simulink model "a8"  (R2021a)
settings: Solver=VariableStepAuto  StartTime=0.0  StopTime=3  RelTol=1e-3
undefined symbols (not defined in the file or in its folder): Down, Ion, Lithium, Up
libraries: spsCurrentMeasurementLib x22, spsVoltageMeasurementLib x17, spsSeriesRLCBranchLib x11, spsGroundLib x6, powerlib_extras x4, spsACVoltageSourceLib x3, spsIGBTDiodeLib x3, dspsigops x3, spsPower3phInstantaneousLib x3, spsDiodeLib x2, spsUniversalBridgeLib x2, spsBatteryLib x1
(part 1 of 2)
settings Model: Creator=Dell  LastModifiedBy=Dell
settings SolverCC: ZeroCrossControl=DisableAll
settings DebuggingCC: ModelReferenceExtraNoncontSigs=none

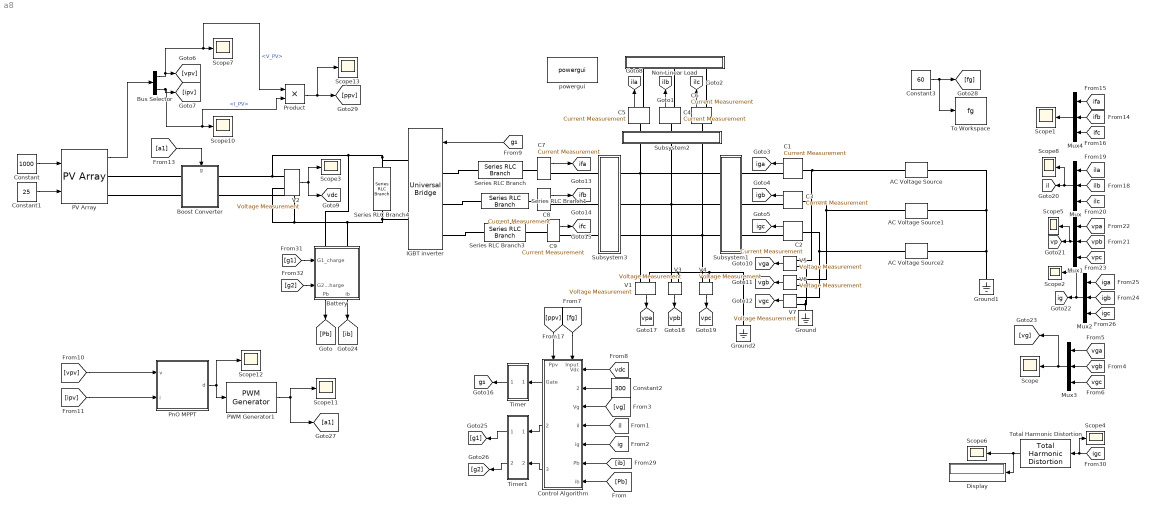
== system a8 ==
  AC Voltage Source : spsACVoltageSourceLib/AC Voltage Source  Amplitude=230  Phase=0  Frequency=60  SampleTime=0  Measurements=None  BusType=swing  Pref=10e3  Qref=0  Qmin=-inf  Qmax=+inf
  AC Voltage Source1 : spsACVoltageSourceLib/AC Voltage Source  Amplitude=230  Phase=120  Frequency=60  SampleTime=0  Measurements=None  BusType=swing  Pref=10e3  Qref=0  Qmin=-inf  Qmax=+inf
  AC Voltage Source2 : spsACVoltageSourceLib/AC Voltage Source  Amplitude=230  Phase=-120  Frequency=60  SampleTime=0  Measurements=None  BusType=swing  Pref=10e3  Qref=0  Qmin=-inf  Qmax=+inf
  Battery : Subsystem
      settings: PortSchema="{\"entries\":[{\"content\":{\"sides\":[{\"content\":{\"connectorIds\":[\"LConn1\",\"LConn2\"]},\"type\":\"ConnectorPlacement.EquallySpacedRectSide\",\"uuid\":\"3f024d4f-4944-46f1-a681-19b9b6f5c2e3\"},{\"content\":{\"connectorIds\":[\"Out1\",\"Out2\"],\"side\":\"RIGHT\"},\"type\":\"ConnectorPlacement.EquallySpacedRectSide\",\"uuid\":\"ba9189b8-b241-4d0f-92c2-ffae32477602\"},{\"content\":{\"connectorIds\":[\"In1\",\"In2\"],\"side\":\"TOP\"},\"type\":\"ConnectorPlacement.EquallySpacedRectSide\",\"uuid\":\"2b5a68b6-4f88-4313-be0a-70c6e84ce948\"}]},\"type\":\"ConnectorPlacement.EquallySpacedConnector\",\"uuid\":\"57f7ac83-2601-4f06-be16-46ca99d36a1f\"}],\"packageUris\":[\"http://schema.mathworks.com/mf0/Connector/R2020b\"],\"version\":\"1.0\"}"
  Boost Converter : Subsystem
      settings: PortSchema="{\"entries\":[{\"content\":{\"sides\":[{\"content\":{\"connectorIds\":[\"LConn1\",\"LConn2\"]},\"type\":\"ConnectorPlacement.EquallySpacedRectSide\",\"uuid\":\"8d150eef-90b5-4fdb-be84-a9f6f4ebd895\"},{\"content\":{\"connectorIds\":[\"RConn1\",\"RConn2\"],\"side\":\"RIGHT\"},\"type\":\"ConnectorPlacement.EquallySpacedRectSide\",\"uuid\":\"8602e169-ea88-4412-9b25-fadbb117dfcf\"},{\"content\":{\"connectorIds\":[\"In1\"],\"side\":\"TOP\"},\"type\":\"ConnectorPlacement.EquallySpacedRectSide\",\"uuid\":\"8809c1af-ab1c-4eed-b81f-f8f2792471ea\"}]},\"type\":\"ConnectorPlacement.EquallySpacedConnector\",\"uuid\":\"c77f0f7f-21b7-47e6-a535-29cdb02ea9e2\"}],\"packageUris\":[\"http://schema.mathworks.com/mf0/Connector/R2020b\"],\"version\":\"1.0\"}"
  Bus Selector : BusSelector  OutputSignals=V_PV,I_PV
  C{1..9} (9 alike) : spsCurrentMeasurementLib/Current Measurement  PhasorSimulation=off  OutputType=Complex  PSBequivalent=0
  Constant : Constant  Value=1000
  Constant1 : Constant  Value=25
  Constant2 : Constant  Value=300
  Constant3 : Constant  Value=60
  Control Algorithm : Subsystem
      settings: PortSchema="{\"entries\":[{\"content\":{\"sides\":[{\"content\":{\"connectorIds\":[\"In1\",\"In2\",\"In3\",\"In4\",\"In5\",\"In6\",\"In7\"]},\"type\":\"ConnectorPlacement.EquallySpacedRectSide\",\"uuid\":\"49955e1e-2d38-4dcf-bb6a-38e771f1236c\"},{\"content\":{\"connectorIds\":[\"Out1\",\"Out2\",\"Out3\"],\"side\":\"RIGHT\"},\"type\":\"ConnectorPlacement.EquallySpacedRectSide\",\"uuid\":\"694b0366-9509-4aa0-9deb-ec901696235e\"},{\"content\":{\"connectorIds\":[\"In8\",\"In9\"],\"side\":\"TOP\"},\"type\":\"ConnectorPlacement.EquallySpacedRectSide\",\"uuid\":\"46f645d8-58d8-49b1-a06d-69f87343fd2f\"}]},\"type\":\"ConnectorPlacement.EquallySpacedConnector\",\"uuid\":\"9b034317-3015-420d-970f-6f1221e48493\"}],\"packageUris\":[\"http://schema.mathworks.com/mf0/Connector/R2020b\"],\"version\":\"1.0\"}"
  Display : Display
  Ground : spsGroundLib/Ground  LConnTagsString=a
  Ground1 : spsGroundLib/Ground  LConnTagsString=a
  Ground2 : spsGroundLib/Ground  LConnTagsString=a
  IGBT inverter : spsUniversalBridgeLib/Universal Bridge  Arms=3  SnubberResistance=1e5  SnubberCapacitance=inf  Device=IGBT / Diodes  Ron=1e-3  Lon=0  ForwardVoltages="[  0  0  ]"  ForwardVoltage=0  GTOparameters=[ 10e-6 , 20e-6 ]  IGBTparameters=[ 1e-6 , 2e-6 ]  Measurements=Device voltages  Measurements_2=None  converterType=Rectifier
  Mux{,1..4} (5 alike) : Mux  Inputs=3
  Non-Linear Load : Subsystem
  PV Array : spsPVArrayLib/PV Array  Npar=1  Nser=6  PlotType=array @ 1000 W/m2 & specified temperatures  S_vec="[ 1000  500  100 ]"  Temp_C_vec="[ 25  ]"  ModuleName=User-defined  PlotWhenSelected=off  Pm=335.28  Ncell=60  Voc=46.8  Isc=9.3  Vm=38.1  Im=8.8  beta_Voc_pc=-0.36099  alpha_Isc_pc=0.102  beta_Voc=-0.16894  alpha_Isc=0.009486  IL=9.3302  I0=3.4457e-10  nI=1.2642  Rsh=710.4206  Rs=0.33548  RobustModel=off  RobustCellTemperature=313.3991  BAL=on  Tc=1e-6  Tfilter=5e-5
  PWM Generator1 : eePwmGenerator/PWM Generator  CarrCount=Up-Down  Tper=1/10000  Ts=5e-6
  PnO MPPT : MATLAB Function  TreatAsAtomicUnit=on
  Product : Product
  Scope{,1..8,10..13} (13 alike) : Scope
  Series RLC Branch : spsSeriesRLCBranchLib/Series RLC Branch  LConnTagsString=__new0  RConnTagsString=__new0  BranchType=L  Resistance=1  Inductance=5e-3  SetiL0=off  InitialCurrent=0  Capacitance=1e-6  Setx0=off  InitialVoltage=0  Measurements=None
  Series RLC Branch1 : spsSeriesRLCBranchLib/Series RLC Branch  LConnTagsString=__new0  RConnTagsString=__new0  BranchType=L  Resistance=1  Inductance=5e-3  SetiL0=off  InitialCurrent=0  Capacitance=1e-6  Setx0=off  InitialVoltage=0  Measurements=None
  Series RLC Branch3 : spsSeriesRLCBranchLib/Series RLC Branch  LConnTagsString=__new0  RConnTagsString=__new0  BranchType=L  Resistance=1  Inductance=5e-3  SetiL0=off  InitialCurrent=0  Capacitance=1e-6  Setx0=off  InitialVoltage=0  Measurements=None
  Series RLC Branch4 : spsSeriesRLCBranchLib/Series RLC Branch  LConnTagsString=__new0  RConnTagsString=__new0  BranchType=C  Resistance=1  Inductance=5e-3  SetiL0=off  InitialCurrent=0  Capacitance=1100e-6  Setx0=off  InitialVoltage=300  Measurements=None
  Subsystem1 : Subsystem
  Subsystem2 : Subsystem
  Subsystem3 : Subsystem
  Timer : Subsystem
  Timer1 : Subsystem
  To Workspace : ToWorkspace  VariableName=fg  SampleTime=-1
      settings: Save2DSignal=2-D array (concatenate along first dimension)
  Total Harmonic Distortion : eeTotalHarmonicDistorsion/Total Harmonic Distortion  f=50  Ts=-1
      settings: SourceProductBaseCode=PS
  V{1..7} (7 alike) : spsVoltageMeasurementLib/Voltage Measurement  PhasorSimulation=off  OutputType=Complex  PSBequivalent=0
  powergui : spspowerguiLib/powergui  Priority=1  SimulationMode=Discrete  SampleTime=5e-6  frequency=60  Iterations=50  frequencyindice=0  Pbase=100e6  ErrMax=1e-4  UnitsV=kV  UnitsW=MW  buscounter=0  FunctionMessages=off  echomessages=off  EnableUseOfTLC=off  CurrentSourceSwitches=off  DisableSnubberDevices=off  DisableRonSwitches=off  DisableVfSwitches=off  DisplayEquations=off  AutomaticDiscreteSolvers=off  SolverType=Tustin/Backward Euler (TBE)  Interpol=off  ExternalGateDelay=off  methode=off  Ts=100  x0status=blocks  SPID=on  SwTol=0  HookPort=off  NonlinearTolerance=1e-4  nMaxIteration=100  ContinueOnMaxIteration=off  RestoreLinks=warning  ResistiveCurrentMeasurement=off  Frange=[0:2:500]  Ylog=off  Xlog=on  ShowGrid=off  save=off  variable=ZData  structure=0  ZoomFFT=off  StartTime=0.0  cycles=1  DisplayStyle=1  fundamental=60  FreqAxis=off  MaxFrequency=1000  frequencyindicesteady=1  RmsSteady=1  display=off
  tag scope: gs=global, ifa=global, ifb=global, ifc=global, ig=global, iga=global, igb=global, igc=global, il=global, ila=global, ilb=global, ilc=global, vdc=global, vga=global, vgb=global, vgc=global, vp=global, vpa=global, vpb=global, vpc=global
  wires:
  Constant/1 -> PV Array/1
  Constant1/1 -> PV Array/2
  V2/1 -> [vdc], Scope3/1
  [g2] -> Battery/2(G2_discharge)
  Battery/2(ib) -> [ib]
  [g1] -> Battery/1(G1_charge)
  Battery/1(Pb) -> [Pb]
  V3/1 -> [vpb]
  V1/1 -> [vpa]
  V4/1 -> [vpc]
  V7/1 -> [vgc]
  V5/1 -> [vga]
  V6/1 -> [vgb]
  C1/1 -> [iga]
  C3/1 -> [igb]
  C2/1 -> [igc]
  [vgb] -> Mux3/2
  Mux3/1 -> [vg], Scope/1
  [vga] -> Mux3/1
  [vgc] -> Mux3/3
  Mux4/1 -> Scope1/1
  Total Harmonic Distortion/1 -> Scope6/1, Display/1
  [ila] -> Mux/1
  [ilb] -> Mux/2
  [vpc] -> Mux1/3
  [ifc] -> Mux4/3
  [iga] -> Mux2/1
  [ilc] -> Mux/3
  [vpa] -> Mux1/1
  Mux2/1 -> Scope2/1, [ig]
  [igb] -> Mux2/2
  Mux1/1 -> Scope5/1, [vp]
  [vpb] -> Mux1/2
  Mux/1 -> [il], Scope8/1
  [ifa] -> Mux4/1
  [igc] -> Scope4/1, Total Harmonic Distortion/1
  [igc] -> Mux2/3
  [ifb] -> Mux4/2
  C7/1 -> [ifa]
  C8/1 -> [ifb]
  C9/1 -> [ifc]
  [vdc] -> Control Algorithm/1(Vdc)
  Timer1/2(g2) -> [g2]
  Control Algorithm/3(gate3) -> Timer1/2(2)
  [vg] -> Control Algorithm/3(Vg)
  [ib] -> Control Algorithm/6(Pb)
  Timer/1(Out1) -> [gs]
  Timer1/1(g1) -> [g1]
  [il] -> Control Algorithm/4(il)
  Control Algorithm/1(Gate) -> Timer/1(In1)
  Control Algorithm/2(gate2) -> Timer1/1(In1)
  [ig] -> Control Algorithm/5(ig)
  Constant2/1 -> Control Algorithm/2(Vdcref)
  [gs] -> IGBT inverter/1
  C4/1 -> [ilb]
  C6/1 -> [ilc]
  Product/1 -> Scope13/1, [ppv]
  PV Array/1 -> Bus Selector/1
  Bus Selector/1 -> Product/1, Scope7/1, [vpv]  "<V_PV>"
  Bus Selector/2 -> Product/2, Scope10/1, [ipv]  "<I_PV>"
  C5/1 -> [ila]
  [a1] -> Boost Converter/1(g)
  PnO MPPT/1(d) -> Scope12/1, PWM Generator1/1
  PWM Generator1/1 -> Scope11/1, [a1]
  [vpv] -> PnO MPPT/1(v)
  [ipv] -> PnO MPPT/2(i)
  [Pb] -> Control Algorithm/7(ib)
  Constant3/1 -> To Workspace/1, [fg]
  [fg] -> Control Algorithm/8(Input)
  [ppv] -> Control Algorithm/9(Ppv)
  connections:
  Boost Converter/LConn1 -- PV Array/RConn1
  Boost Converter/LConn2 -- PV Array/RConn2
  Boost Converter/RConn1 -- Battery/LConn1 -- Series RLC Branch4/LConn1 -- IGBT inverter/RConn1 -- V2/LConn1
  Boost Converter/RConn2 -- Series RLC Branch4/RConn1 -- IGBT inverter/RConn2 -- Battery/LConn2 -- V2/LConn2
  Series RLC Branch3/LConn1 -- IGBT inverter/LConn3
  Series RLC Branch1/LConn1 -- IGBT inverter/LConn2
  Series RLC Branch/LConn1 -- IGBT inverter/LConn1
  Ground2/LConn1 -- V1/LConn2 -- V3/LConn2 -- V4/LConn2
  V7/LConn2 -- Ground/LConn1 -- V5/LConn2 -- V6/LConn2
  C3/LConn1 -- AC Voltage Source1/RConn1 -- V6/LConn1
  Subsystem3/LConn2 -- C8/RConn1
  Subsystem3/LConn1 -- C7/RConn1
  Subsystem3/LConn3 -- C9/RConn1
  Subsystem3/RConn1 -- V1/LConn1 -- Subsystem2/LConn1 -- Subsystem1/RConn1
  Subsystem3/RConn2 -- V3/LConn1 -- Subsystem2/LConn2 -- Subsystem1/RConn2
  Subsystem3/RConn3 -- V4/LConn1 -- Subsystem2/LConn3 -- Subsystem1/RConn3
  Subsystem1/LConn1 -- C1/RConn1
  Subsystem1/LConn2 -- C3/RConn1
  C2/RConn1 -- Subsystem1/LConn3
  C7/LConn1 -- Series RLC Branch/RConn1
  C8/LConn1 -- Series RLC Branch1/RConn1
  C9/LConn1 -- Series RLC Branch3/RConn1
  Non-Linear Load/LConn2 -- C4/RConn1
  C4/LConn1 -- Subsystem2/RConn2
  C5/LConn1 -- Subsystem2/RConn1
  Non-Linear Load/LConn3 -- C6/RConn1
  Non-Linear Load/LConn1 -- C5/RConn1
  Subsystem2/RConn3 -- C6/LConn1
  C2/LConn1 -- AC Voltage Source2/RConn1 -- V7/LConn1
  C1/LConn1 -- AC Voltage Source/RConn1 -- V5/LConn1
  AC Voltage Source/LConn1 -- AC Voltage Source1/LConn1 -- AC Voltage Source2/LConn1 -- Ground1/LConn1

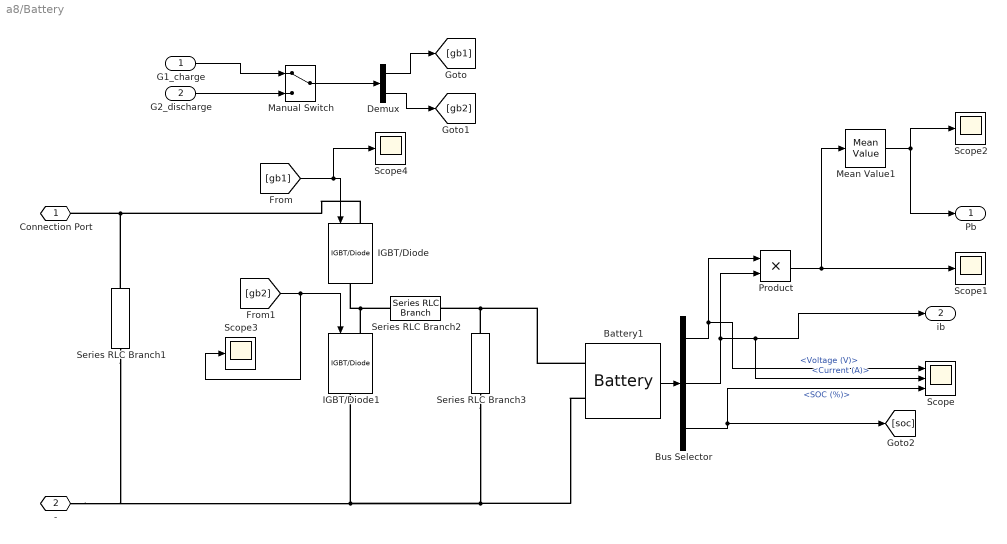
== system a8/Battery ==
  G1_charge : Inport
  G2_discharge : Inport  Port=2
  Battery1 : spsBatteryLib/Battery  BatType=Lithium-Ion  ShowTempParam=off  ThermalPreset=no  ShowAgeParam=off  NomV=72  NomQ=30  SOC=9  Batt_Tr=1  PresetModel=off  MaxQ=30  MinV=54  FullV=83.8071  Dis_rate=8  R=0.024  Normal_OP=27.1304  expZone="[77.7878      1.47391]"  current=[6.5 13 32.5]  Units=Time  Tci=20  NomT=20  T2=-30  MaxQ2=4.8  FullV2=7.1  Normal_OP2=5.655  expZone2="[6.58           1]"  Rca=0.6  ti=2000  Dp=0  Neq0=0  Tsim=1e6  Ta1=25  Qeol=5.4*0.9  Reol=0.013333*1.2  Char_age=[2.3478, 3]  Dis_age=[2.3478, 10]  N1=1500  N2=10500  N3=1000  N4=1400  Ta2=45  N5=950
  Bus Selector : BusSelector  OutputSignals=Voltage (V),Current (A),SOC (%)
  Demux : Demux  Outputs=2
  IGBT/Diode : spsIGBTDiodeLib/IGBT//Diode  Ron=1e-3  Rs=1e5  Cs=inf  Measurements=off
  IGBT/Diode1 : spsIGBTDiodeLib/IGBT//Diode  Ron=1e-3  Rs=1e5  Cs=inf  Measurements=off
  Manual Switch : ManualSwitch
  Mean Value1 : powerlib_extras/Measurements/Mean Value  Period=1/100
      settings: SourceProductBaseCode=PS
  Product : Product
  Scope : Scope  NumInputPorts=3
  Scope{1..4} (4 alike) : Scope
  Series RLC Branch1 : spsSeriesRLCBranchLib/Series RLC Branch  LConnTagsString=__new0  RConnTagsString=__new0  BranchType=C  Resistance=1  Inductance=1e-3  SetiL0=off  InitialCurrent=0  Capacitance=1100e-6  Setx0=off  InitialVoltage=0  Measurements=None
  Series RLC Branch2 : spsSeriesRLCBranchLib/Series RLC Branch  LConnTagsString=__new0  RConnTagsString=__new0  BranchType=L  Resistance=1  Inductance=2e-3  SetiL0=off  InitialCurrent=0  Capacitance=1e-6  Setx0=off  InitialVoltage=0  Measurements=None
  Series RLC Branch3 : spsSeriesRLCBranchLib/Series RLC Branch  LConnTagsString=__new0  RConnTagsString=__new0  BranchType=C  Resistance=1  Inductance=1e-3  SetiL0=off  InitialCurrent=0  Capacitance=1100e-6  Setx0=off  InitialVoltage=0  Measurements=None
  Connection Port : PMIOPort  Side=Left
  - : PMIOPort  Port=2  Side=Left
  Pb : Outport
  ib : Outport  Port=2
  wires:
  Battery1/1 -> Bus Selector/1
  Bus Selector/1 -> Product/1, Scope/1  "<Voltage (V)>"
  Bus Selector/2 -> ib/1, Scope/2, Product/2  "<Current (A)>"
  Product/1 -> Mean Value1/1, Scope1/1
  Bus Selector/3 -> Scope/3, [soc]  "<SOC (%)>"
  Mean Value1/1 -> Scope2/1, Pb/1
  [gb1] -> Scope4/1, IGBT/Diode/1
  [gb2] -> Scope3/1, IGBT/Diode1/1
  Demux/1 -> [gb1]
  Demux/2 -> [gb2]
  Manual Switch/1 -> Demux/1
  G1_charge/1 -> Manual Switch/1
  G2_discharge/1 -> Manual Switch/2
  connections:
  Battery1/LConn1 -- Series RLC Branch3/LConn1 -- Series RLC Branch2/RConn1
  IGBT/Diode1/LConn1 -- Series RLC Branch2/LConn1 -- IGBT/Diode/RConn1
  Series RLC Branch3/RConn1 -- Series RLC Branch1/RConn1 -- -/RConn1 -- IGBT/Diode1/RConn1 -- Battery1/LConn2
  IGBT/Diode/LConn1 -- Series RLC Branch1/LConn1 -- Connection Port/RConn1

== system a8/Boost Converter ==
  g : Inport
  Diode1 : spsDiodeLib/Diode  Ron=0.001  Lon=0  Vf=0.8  IC=0  UseSnubber=0  Rs=0  Cs=0  Measurements=off
  Diode2 : spsDiodeLib/Diode  Ron=0.001  Lon=0  Vf=0.8  IC=0  UseSnubber=0  Rs=0  Cs=0  Measurements=off
  IGBT/Diode : spsIGBTDiodeLib/IGBT//Diode  Ron=1e-3  Rs=1e5  Cs=inf  Measurements=off
  Series RLC Branch : spsSeriesRLCBranchLib/Series RLC Branch  LConnTagsString=__new0  RConnTagsString=__new0  BranchType=L  Resistance=1  Inductance=5e-3  SetiL0=off  InitialCurrent=0  Capacitance=1e-6  Setx0=off  InitialVoltage=0  Measurements=None
  Series RLC Branch1 : spsSeriesRLCBranchLib/Series RLC Branch  LConnTagsString=__new0  RConnTagsString=__new0  BranchType=C  Resistance=1  Inductance=1e-3  SetiL0=off  InitialCurrent=0  Capacitance=1100e-6  Setx0=off  InitialVoltage=0  Measurements=None
  Series RLC Branch2 : spsSeriesRLCBranchLib/Series RLC Branch  LConnTagsString=__new0  RConnTagsString=__new0  BranchType=C  Resistance=1  Inductance=1e-3  SetiL0=off  InitialCurrent=0  Capacitance=1100e-6  Setx0=off  InitialVoltage=0  Measurements=None
  1 : PMIOPort  Side=Left
  Connection Port : PMIOPort  Port=2  Side=Left
  Connection Port1 : PMIOPort  Port=3  Side=Right
  Connection Port2 : PMIOPort  Port=4  Side=Right
  wires:
  g/1 -> IGBT/Diode/1
  connections:
  IGBT/Diode/LConn1 -- Series RLC Branch/RConn1 -- Diode2/LConn1
  Diode2/RConn1 -- Diode1/LConn1 -- Series RLC Branch2/LConn1
  Series RLC Branch/LConn1 -- Series RLC Branch1/LConn1 -- 1/RConn1
  IGBT/Diode/RConn1 -- Connection Port/RConn1 -- Series RLC Branch1/RConn1 -- Connection Port2/RConn1 -- Series RLC Branch2/RConn1
  Connection Port1/RConn1 -- Diode1/RConn1

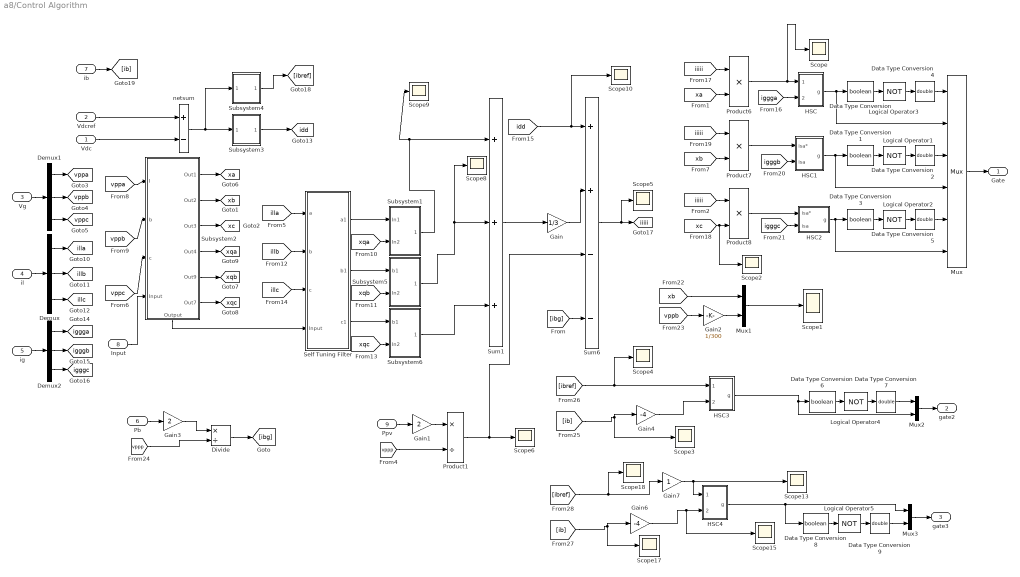
== system a8/Control Algorithm ==
  Vdc : Inport
  Vdcref : Inport  Port=2
  Vg : Inport  Port=3
  il : Inport  Port=4
  ig : Inport  Port=5
  Pb : Inport  Port=6
  ib : Inport  Port=7
  Input : Inport  Port=8
  Ppv : Inport  Port=9
  Data Type Conversion{,1,3,6,8} (5 alike) : DataTypeConversion  OutDataTypeStr=boolean  SaturateOnIntegerOverflow=on  RndMeth=Zero
  Data Type Conversion{2,4..5,7,9} (5 alike) : DataTypeConversion  OutDataTypeStr=double  SaturateOnIntegerOverflow=on  RndMeth=Zero
  Demux : Demux  Outputs=3
  Demux1 : Demux  Outputs=3
  Demux2 : Demux  Outputs=3
  Divide : Product  Inputs=*/
  Gain : Gain  Gain=1/3
  Gain1 : Gain  Gain=2
  Gain2 : Gain  Gain=1/300
  Gain3 : Gain  Gain=2
  Gain4 : Gain  Gain=-4
  Gain6 : Gain  Gain=-4
  Gain7 : Gain
  HSC : Subsystem  mask{h=.005}
      mask prompts: h "Hysteresis band (A)"
      mask help: Hysteresis Current Controller
      mask Display: plot(0,0,100,100,[45,45],[35,65],[55,55],[35,65],[45,65],[65,65],[35,55],[35,35])
  HSC1 : Subsystem  mask{h=.005}
      mask prompts: h "Hysteresis band (A)"
      mask help: Hysteresis Current Controller
      mask Display: plot(0,0,100,100,[45,45],[35,65],[55,55],[35,65],[45,65],[65,65],[35,55],[35,35])
  HSC2 : Subsystem  mask{h=.005}
      mask prompts: h "Hysteresis band (A)"
      mask help: Hysteresis Current Controller
      mask Display: plot(0,0,100,100,[45,45],[35,65],[55,55],[35,65],[45,65],[65,65],[35,55],[35,35])
  HSC3 : Subsystem  mask{h=.005}
      mask prompts: h "Hysteresis band (A)"
      mask help: Hysteresis Current Controller
      mask Display: plot(0,0,100,100,[45,45],[35,65],[55,55],[35,65],[45,65],[65,65],[35,55],[35,35])
  HSC4 : Subsystem  mask{h=.005}
      mask prompts: h "Hysteresis band (A)"
      mask help: Hysteresis Current Controller
      mask Display: plot(0,0,100,100,[45,45],[35,65],[55,55],[35,65],[45,65],[65,65],[35,55],[35,35])
  Logical Operator{1..5} (5 alike) : Logic  Operator=NOT  AllPortsSameDT=off  OutDataTypeStr=boolean
  Mux : Mux  Inputs=6
  Mux1 : Mux  Inputs=2
  Mux2 : Mux  Inputs=2
  Mux3 : Mux  Inputs=2
  Product1 : Product  Inputs=*/  RndMeth=Zero
  Product6 : Product  RndMeth=Zero
  Product7 : Product  RndMeth=Zero
  Product8 : Product  RndMeth=Zero
  Scope{,1..6,8..10,13,15,17..18} (14 alike) : Scope
  Self Tuning Filter : Subsystem
  Subsystem1 : Subsystem
  Subsystem2 : Subsystem
      settings: PortSchema="{\"entries\":[{\"content\":{\"sides\":[{\"content\":{\"connectorIds\":[\"In1\",\"In2\",\"In3\",\"In4\"]},\"type\":\"ConnectorPlacement.EquallySpacedRectSide\",\"uuid\":\"d21a8900-8593-46dc-a973-eb44ab28bf11\"},{\"content\":{\"connectorIds\":[\"Out1\",\"Out2\",\"Out3\",\"Out4\",\"Out5\",\"Out6\"],\"side\":\"RIGHT\"},\"type\":\"ConnectorPlacement.EquallySpacedRectSide\",\"uuid\":\"7b79a857-e0e8-4093-8398-4f53d30614a1\"},{\"content\":{\"connectorIds\":[],\"side\":\"TOP\"},\"type\":\"ConnectorPlacement.EquallySpacedRectSide\",\"uuid\":\"19a1b9b6-80af-4e74-b995-bbf8c7c9712f\"},{\"content\":{\"connectorIds\":[\"Out7\"],\"side\":\"BOTTOM\"},\"type\":\"ConnectorPlacement.EquallySpacedRectSide\",\"uuid\":\"3e15eaf6-e5fa-4fbd-8cf9-a9cde768b274\"}]},\"type\":\"ConnectorPlacement.EquallySpacedConnector\",\"uuid\":\"e55638c6-9abc-4009-b2e0-3c40bc063c83\"}],\"packageUris\":[\"http://schema.mathworks.com/mf0/Connector/R2020b\"],\"version\":\"1.0\"}"
  Subsystem3 : Subsystem
  Subsystem4 : Subsystem
  Subsystem5 : Subsystem
  Subsystem6 : Subsystem
  Sum1 : Sum  Inputs=+++  InputSameDT=on  SaturateOnIntegerOverflow=on  OutDataTypeStr=Inherit: Same as first input
  Sum6 : Sum  Inputs=++--  InputSameDT=on  SaturateOnIntegerOverflow=on  OutDataTypeStr=Inherit: Same as first input
  netsum : Sum  Inputs=+-  InputSameDT=on  SaturateOnIntegerOverflow=on  OutDataTypeStr=Inherit: Same as first input
  Gate : Outport
  gate2 : Outport  Port=2
  gate3 : Outport  Port=3
  tag scope: idd=global, iggga=global, igggb=global, igggc=global, iiiii=global, illa=global, illb=global, illc=global, vppa=global, vppb=global, vppc=global, xa=global, xb=global, xc=global, xqa=global, xqb=global, xqc=global
  wires:
  netsum/1 -> Subsystem4/1(In1), Subsystem3/1(In1)
  Subsystem2/3(Out3) -> [xc]
  Subsystem2/2(Out2) -> [xb]
  Subsystem2/1(Out1) -> [xa]
  [xa] -> Product6/2
  [xb] -> Product7/2
  [xc] -> Scope2/1, Product8/2
  HSC/1(g) -> Mux/2, Data Type Conversion/1
  Mux/1 -> Gate/1
  Product7/1 -> HSC1/1(isa*)
  Product8/1 -> HSC2/1(isa*)
  Data Type Conversion/1 -> Logical Operator3/1
  Logical Operator3/1 -> Data Type Conversion4/1
  Data Type Conversion4/1 -> Mux/1
  HSC1/1(g) -> Mux/4, Data Type Conversion1/1
  Data Type Conversion1/1 -> Logical Operator1/1
  Logical Operator1/1 -> Data Type Conversion2/1
  Data Type Conversion2/1 -> Mux/3
  Data Type Conversion3/1 -> Logical Operator2/1
  Logical Operator2/1 -> Data Type Conversion5/1
  Data Type Conversion5/1 -> Mux/5
  HSC2/1(g) -> Mux/6, Data Type Conversion3/1
  Ppv/1 -> Gain1/1
  Gain1/1 -> Product1/1
  [vppp] -> Product1/2
  Product1/1 -> Sum6/3, Scope6/1
  Subsystem3/1(Out1) -> [idd]
  il/1 -> Demux/1
  Vg/1 -> Demux1/1
  ig/1 -> Demux2/1
  Demux1/1 -> [vppa]
  Demux1/2 -> [vppb]
  Demux1/3 -> [vppc]
  [vppa] -> Subsystem2/1(I)
  [vppb] -> Subsystem2/2(b)
  [vppc] -> Subsystem2/3(c)
  Subsystem2/4(Out4) -> [xqa]
  Subsystem2/5(Out9) -> [xqb]
  Subsystem2/6(Out7) -> [xqc]
  Demux/3 -> [illc]
  Demux/2 -> [illb]
  Demux/1 -> [illa]
  Subsystem1/1(Out1) -> Scope9/1, Sum1/1
  Subsystem5/1(Out1) -> Scope8/1, Sum1/2
  Subsystem6/1(Out1) -> Sum1/3
  Demux2/1 -> [iggga]
  Demux2/2 -> [igggb]
  Demux2/3 -> [igggc]
  Sum6/1 -> Scope5/1, [iiiii]
  [iiiii] -> Product7/1
  [iiiii] -> Product6/1
  [iiiii] -> Product8/1
  [iggga] -> HSC/2(isa)
  [igggb] -> HSC1/2(isa)
  [igggc] -> HSC2/2(isa)
  [xb] -> Mux1/1
  [vppb] -> Gain2/1
  Mux1/1 -> Scope1/1
  Gain2/1 -> Mux1/2
  Vdcref/1 -> netsum/1
  Product6/1 -> Scope/1, HSC/1(isa*)
  Vdc/1 -> netsum/2
  Sum1/1 -> Gain/1
  Gain/1 -> Sum6/2
  Pb/1 -> Gain3/1
  Gain3/1 -> Divide/1
  [vppp] -> Divide/2
  Divide/1 -> [ibg]
  [ibg] -> Sum6/4
  ib/1 -> [ib]
  [ibref] -> Scope4/1, HSC3/1(isa*)
  Logical Operator4/1 -> Data Type Conversion7/1
  Data Type Conversion6/1 -> Logical Operator4/1
  HSC3/1(g) -> Mux2/2, Data Type Conversion6/1
  Data Type Conversion7/1 -> Mux2/1
  Mux2/1 -> gate2/1
  [ib] -> Gain4/1, Scope3/1
  Gain4/1 -> HSC3/2(isa)
  Subsystem4/1(Out1) -> [ibref]
  [illb] -> Self Tuning Filter/2(b)
  Self Tuning Filter/2(b1) -> Subsystem5/1(b1)
  [illa] -> Self Tuning Filter/1(a)
  [illc] -> Self Tuning Filter/3(c)
  Self Tuning Filter/1(a1) -> Subsystem1/1(In1)
  [xqa] -> Subsystem1/2(In2)
  [xqb] -> Subsystem5/2(In2)
  Self Tuning Filter/3(c1) -> Subsystem6/1(b1)
  [xqc] -> Subsystem6/2(In2)
  Mux3/1 -> gate3/1
  Gain7/1 -> Scope13/1, HSC4/1(isa*)
  Gain6/1 -> Scope15/1, HSC4/2(isa)
  Data Type Conversion8/1 -> Logical Operator5/1
  HSC4/1(g) -> Data Type Conversion8/1, Mux3/1
  [ib] -> Gain6/1, Scope17/1
  Data Type Conversion9/1 -> Mux3/2
  Logical Operator5/1 -> Data Type Conversion9/1
  [ibref] -> Scope18/1, Gain7/1
  Input/1 -> Subsystem2/4(Input)
  Subsystem2/7(Output) -> Self Tuning Filter/4(Input)
  [idd] -> Scope10/1, Sum6/1

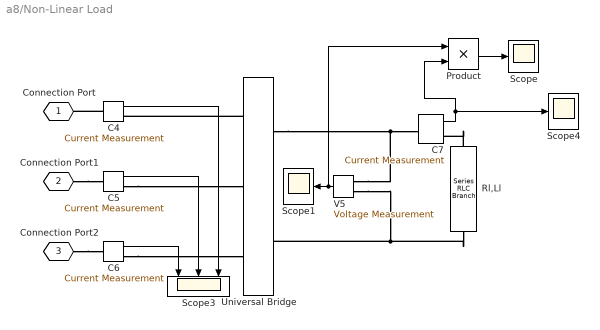
== system a8/Non-Linear Load ==
  C{4..7} (4 alike) : spsCurrentMeasurementLib/Current Measurement  PhasorSimulation=off  OutputType=Complex  PSBequivalent=0
  Product : Product
  Rl,Ll : spsSeriesRLCBranchLib/Series RLC Branch  LConnTagsString=__new0  RConnTagsString=__new0  BranchType=RL  Resistance=200  Inductance=25e-3  SetiL0=off  InitialCurrent=0  Capacitance=1.0  Setx0=off  InitialVoltage=0  Measurements=None
  Scope : Scope
  Scope1 : Scope
  Scope3 : Scope  NumInputPorts=3
  Scope4 : Scope
  Universal Bridge : spsUniversalBridgeLib/Universal Bridge  Arms=3  SnubberResistance=500  SnubberCapacitance=.1e-6  Device=Diodes  Ron=1e-3  Lon=0  ForwardVoltages="[  0  0  ]"  ForwardVoltage=.8  GTOparameters=[ 10e-6 , 20e-6 ]  IGBTparameters=[ 1e-6 , 2e-6 ]  Measurements=Device voltages  Measurements_2=None  converterType=Rectifier
  V5 : spsVoltageMeasurementLib/Voltage Measurement  PhasorSimulation=off  OutputType=Complex  PSBequivalent=0
  Connection Port : PMIOPort  Tag=PMCPort  Side=Left
  Connection Port1 : PMIOPort  Tag=PMCPort  Port=2  Side=Left
  Connection Port2 : PMIOPort  Tag=PMCPort  Port=3  Side=Left
  wires:
  C7/1 -> Product/2, Scope4/1
  V5/1 -> Product/1, Scope1/1
  C6/1 -> Scope3/1
  C5/1 -> Scope3/2
  C4/1 -> Scope3/3
  Product/1 -> Scope/1
  connections:
  Universal Bridge/RConn1 -- V5/LConn1 -- C7/LConn1
  Rl,Ll/LConn1 -- C7/RConn1
  Rl,Ll/RConn1 -- V5/LConn2 -- Universal Bridge/RConn2
  C4/LConn1 -- Connection Port/RConn1
  Connection Port2/RConn1 -- C6/LConn1
  Connection Port1/RConn1 -- C5/LConn1
  C6/RConn1 -- Universal Bridge/LConn3
  C5/RConn1 -- Universal Bridge/LConn2
  Universal Bridge/LConn1 -- C4/RConn1

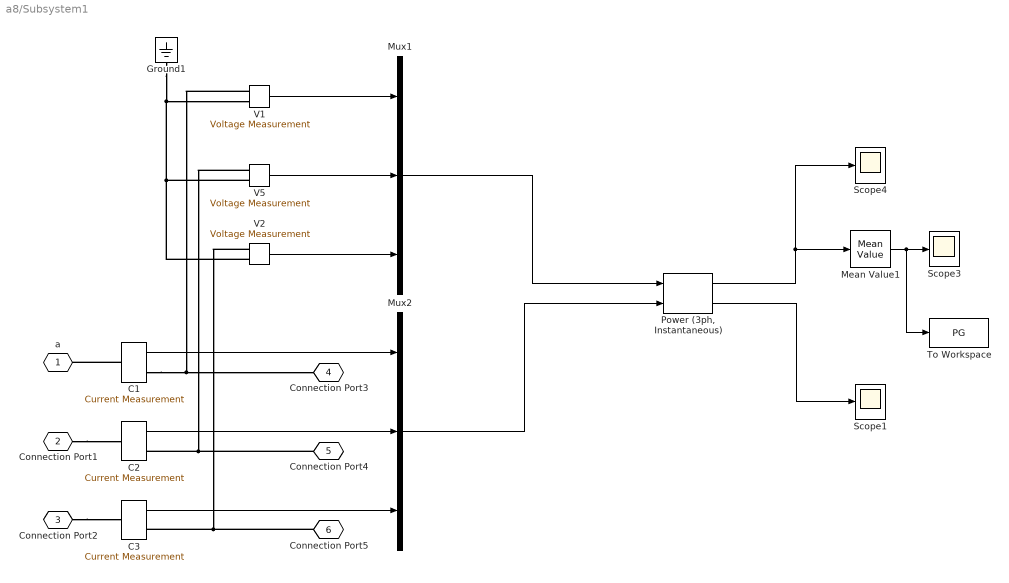
== system a8/Subsystem1 ==
  C1 : spsCurrentMeasurementLib/Current Measurement  PhasorSimulation=off  OutputType=Complex  PSBequivalent=0
  C2 : spsCurrentMeasurementLib/Current Measurement  PhasorSimulation=off  OutputType=Complex  PSBequivalent=0
  C3 : spsCurrentMeasurementLib/Current Measurement  PhasorSimulation=off  OutputType=Complex  PSBequivalent=0
  Ground1 : spsGroundLib/Ground  LConnTagsString=a
  Mean Value1 : powerlib_extras/Measurements/Mean Value  Period=1/100
      settings: SourceProductBaseCode=PS
  Mux1 : Mux  Inputs=3
  Mux2 : Mux  Inputs=3
  "Power (3ph, Instantaneous)" : spsPower3phInstantaneousLib/Power (3ph, Instantaneous)
  Scope1 : Scope
  Scope3 : Scope
  Scope4 : Scope
  To Workspace : ToWorkspace  VariableName=PG  SampleTime=-1
      settings: MaxDataPoints=614863
  V1 : spsVoltageMeasurementLib/Voltage Measurement  PhasorSimulation=off  OutputType=Complex  PSBequivalent=0
  V2 : spsVoltageMeasurementLib/Voltage Measurement  PhasorSimulation=off  OutputType=Complex  PSBequivalent=0
  V5 : spsVoltageMeasurementLib/Voltage Measurement  PhasorSimulation=off  OutputType=Complex  PSBequivalent=0
  a : PMIOPort  Tag=PMCPort  Side=Left
  Connection Port1 : PMIOPort  Tag=PMCPort  Port=2  Side=Left
  Connection Port2 : PMIOPort  Tag=PMCPort  Port=3  Side=Left
  Connection Port3 : PMIOPort  Tag=PMCPort  Port=4  Side=Right
  Connection Port4 : PMIOPort  Tag=PMCPort  Port=5  Side=Right
  Connection Port5 : PMIOPort  Tag=PMCPort  Port=6  Side=Right
  wires:
  Mean Value1/1 -> To Workspace/1, Scope3/1
  C1/1 -> Mux2/1
  C2/1 -> Mux2/2
  C3/1 -> Mux2/3
  V1/1 -> Mux1/1
  V5/1 -> Mux1/2
  V2/1 -> Mux1/3
  Mux1/1 -> "Power (3ph, Instantaneous)"/1
  Mux2/1 -> "Power (3ph, Instantaneous)"/2
  "Power (3ph, Instantaneous)"/2 -> Scope1/1
  "Power (3ph, Instantaneous)"/1 -> Scope4/1, Mean Value1/1
  connections:
  C1/LConn1 -- a/RConn1
  C3/RConn1 -- Connection Port5/RConn1 -- V2/LConn1
  C2/RConn1 -- Connection Port4/RConn1 -- V5/LConn1
  V1/LConn1 -- C1/RConn1 -- Connection Port3/RConn1
  Ground1/LConn1 -- V1/LConn2 -- V2/LConn2 -- V5/LConn2
  Connection Port2/RConn1 -- C3/LConn1
  Connection Port1/RConn1 -- C2/LConn1

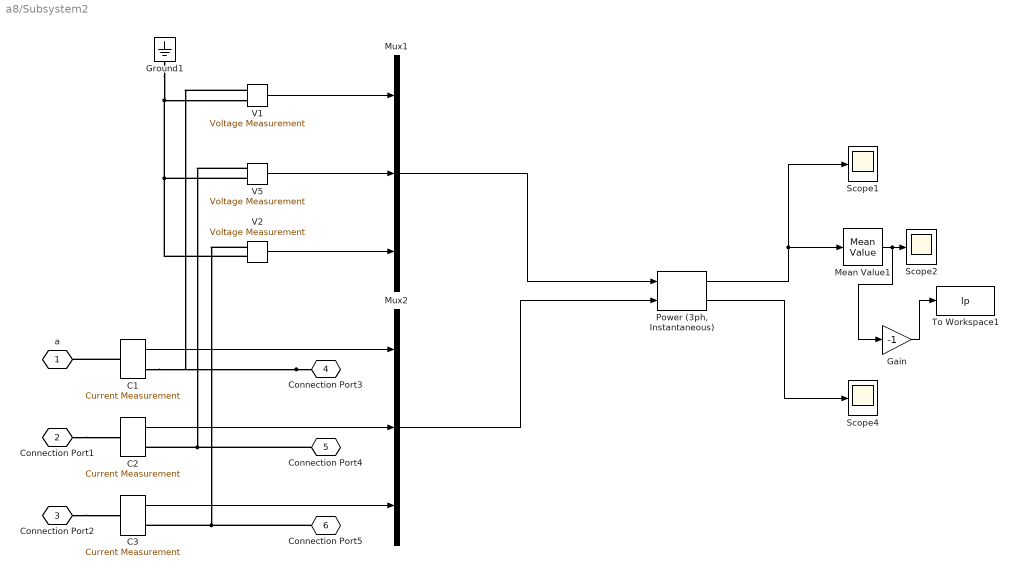
== system a8/Subsystem2 ==
  C1 : spsCurrentMeasurementLib/Current Measurement  PhasorSimulation=off  OutputType=Complex  PSBequivalent=0
  C2 : spsCurrentMeasurementLib/Current Measurement  PhasorSimulation=off  OutputType=Complex  PSBequivalent=0
  C3 : spsCurrentMeasurementLib/Current Measurement  PhasorSimulation=off  OutputType=Complex  PSBequivalent=0
  Gain : Gain  Gain=-1
  Ground1 : spsGroundLib/Ground  LConnTagsString=a
  Mean Value1 : powerlib_extras/Measurements/Mean Value  Period=1/100
      settings: SourceProductBaseCode=PS
  Mux1 : Mux  Inputs=3
  Mux2 : Mux  Inputs=3
  "Power (3ph, Instantaneous)" : spsPower3phInstantaneousLib/Power (3ph, Instantaneous)
  Scope1 : Scope
  Scope2 : Scope
  Scope4 : Scope
  To Workspace1 : ToWorkspace  VariableName=lp  SampleTime=-1
      settings: MaxDataPoints=614863
  V1 : spsVoltageMeasurementLib/Voltage Measurement  PhasorSimulation=off  OutputType=Complex  PSBequivalent=0
  V2 : spsVoltageMeasurementLib/Voltage Measurement  PhasorSimulation=off  OutputType=Complex  PSBequivalent=0
  V5 : spsVoltageMeasurementLib/Voltage Measurement  PhasorSimulation=off  OutputType=Complex  PSBequivalent=0
  a : PMIOPort  Tag=PMCPort  Side=Left
  Connection Port1 : PMIOPort  Tag=PMCPort  Port=2  Side=Left
  Connection Port2 : PMIOPort  Tag=PMCPort  Port=3  Side=Left
  Connection Port3 : PMIOPort  Tag=PMCPort  Port=4  Side=Right
  Connection Port4 : PMIOPort  Tag=PMCPort  Port=5  Side=Right
  Connection Port5 : PMIOPort  Tag=PMCPort  Port=6  Side=Right
  wires:
  "Power (3ph, Instantaneous)"/1 -> Scope1/1, Mean Value1/1
  "Power (3ph, Instantaneous)"/2 -> Scope4/1
  Mux2/1 -> "Power (3ph, Instantaneous)"/2
  Mux1/1 -> "Power (3ph, Instantaneous)"/1
  V2/1 -> Mux1/3
  V5/1 -> Mux1/2
  V1/1 -> Mux1/1
  C3/1 -> Mux2/3
  C2/1 -> Mux2/2
  C1/1 -> Mux2/1
  Mean Value1/1 -> Gain/1, Scope2/1
  Gain/1 -> To Workspace1/1
  connections:
  Connection Port1/RConn1 -- C2/LConn1
  Connection Port2/RConn1 -- C3/LConn1
  V5/LConn2 -- V2/LConn2 -- V1/LConn2 -- Ground1/LConn1
  Connection Port3/RConn1 -- C1/RConn1 -- V1/LConn1
  V5/LConn1 -- Connection Port4/RConn1 -- C2/RConn1
  V2/LConn1 -- Connection Port5/RConn1 -- C3/RConn1
  C1/LConn1 -- a/RConn1

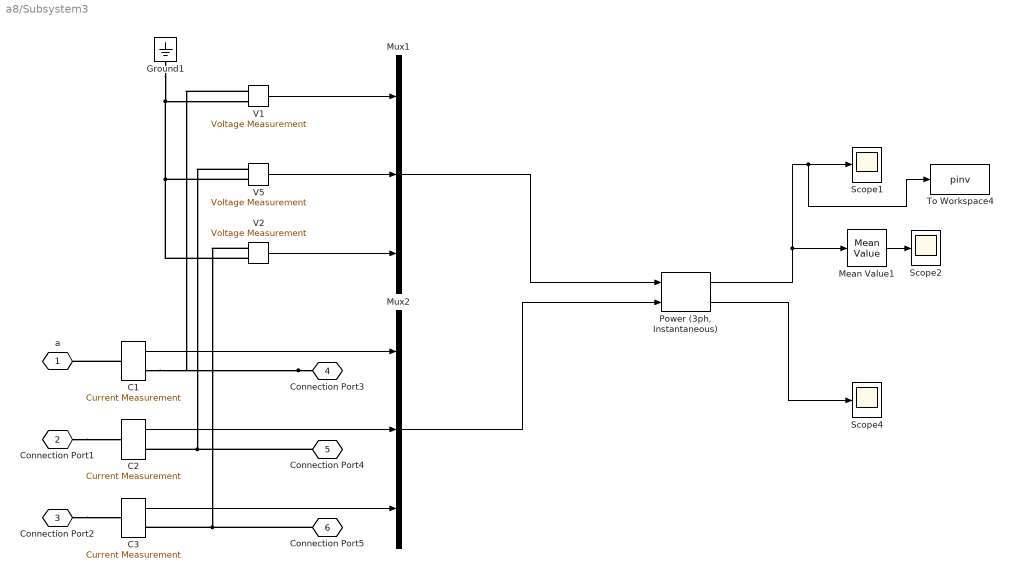
== system a8/Subsystem3 ==
  C1 : spsCurrentMeasurementLib/Current Measurement  PhasorSimulation=off  OutputType=Complex  PSBequivalent=0
  C2 : spsCurrentMeasurementLib/Current Measurement  PhasorSimulation=off  OutputType=Complex  PSBequivalent=0
  C3 : spsCurrentMeasurementLib/Current Measurement  PhasorSimulation=off  OutputType=Complex  PSBequivalent=0
  Ground1 : spsGroundLib/Ground  LConnTagsString=a
  Mean Value1 : powerlib_extras/Measurements/Mean Value  Period=1/100
      settings: SourceProductBaseCode=PS
  Mux1 : Mux  Inputs=3
  Mux2 : Mux  Inputs=3
  "Power (3ph, Instantaneous)" : spsPower3phInstantaneousLib/Power (3ph, Instantaneous)
  Scope1 : Scope
  Scope2 : Scope
  Scope4 : Scope
  To Workspace4 : ToWorkspace  VariableName=pinv  SampleTime=-1
      settings: MaxDataPoints=614863
  V1 : spsVoltageMeasurementLib/Voltage Measurement  PhasorSimulation=off  OutputType=Complex  PSBequivalent=0
  V2 : spsVoltageMeasurementLib/Voltage Measurement  PhasorSimulation=off  OutputType=Complex  PSBequivalent=0
  V5 : spsVoltageMeasurementLib/Voltage Measurement  PhasorSimulation=off  OutputType=Complex  PSBequivalent=0
  a : PMIOPort  Tag=PMCPort  Side=Left
  Connection Port1 : PMIOPort  Tag=PMCPort  Port=2  Side=Left
  Connection Port2 : PMIOPort  Tag=PMCPort  Port=3  Side=Left
  Connection Port3 : PMIOPort  Tag=PMCPort  Port=4  Side=Right
  Connection Port4 : PMIOPort  Tag=PMCPort  Port=5  Side=Right
  Connection Port5 : PMIOPort  Tag=PMCPort  Port=6  Side=Right
  wires:
  "Power (3ph, Instantaneous)"/1 -> To Workspace4/1, Scope1/1, Mean Value1/1
  "Power (3ph, Instantaneous)"/2 -> Scope4/1
  Mux2/1 -> "Power (3ph, Instantaneous)"/2
  Mux1/1 -> "Power (3ph, Instantaneous)"/1
  V2/1 -> Mux1/3
  V5/1 -> Mux1/2
  V1/1 -> Mux1/1
  C3/1 -> Mux2/3
  C2/1 -> Mux2/2
  C1/1 -> Mux2/1
  Mean Value1/1 -> Scope2/1
  connections:
  Connection Port1/RConn1 -- C2/LConn1
  Connection Port2/RConn1 -- C3/LConn1
  V5/LConn2 -- V2/LConn2 -- V1/LConn2 -- Ground1/LConn1
  Connection Port3/RConn1 -- C1/RConn1 -- V1/LConn1
  V5/LConn1 -- Connection Port4/RConn1 -- C2/RConn1
  V2/LConn1 -- Connection Port5/RConn1 -- C3/RConn1
  C1/LConn1 -- a/RConn1

== system a8/Timer ==
  In1 : Inport
  Constant : Constant  Value=0
  Demux : Demux  Outputs=6
  Logical Operator3 : Logic  Operator=NOT  AllPortsSameDT=off  OutDataTypeStr=boolean
  Mux : Mux  Inputs=6
  Step2 : Step  Time=0  SampleTime=0
  Switch{,1..5} (6 alike) : Switch  Criteria=u2 ~= 0
  Out1 : Outport
  wires:
  In1/1 -> Demux/1
  Constant/1 -> Switch1/1, Switch2/1, Switch5/1, Switch4/1, Switch3/1, Switch/1
  Demux/6 -> Switch5/3
  Demux/5 -> Switch4/3
  Demux/4 -> Switch3/3
  Demux/3 -> Switch2/3
  Demux/2 -> Switch1/3
  Demux/1 -> Switch/3
  Step2/1 -> Logical Operator3/1
  Switch/1 -> Mux/1
  Switch1/1 -> Mux/2
  Switch2/1 -> Mux/3
  Switch3/1 -> Mux/4
  Switch4/1 -> Mux/5
  Switch5/1 -> Mux/6
  Mux/1 -> Out1/1
  Logical Operator3/1 -> Switch3/2, Switch5/2, Switch4/2, Switch/2, Switch1/2, Switch2/2

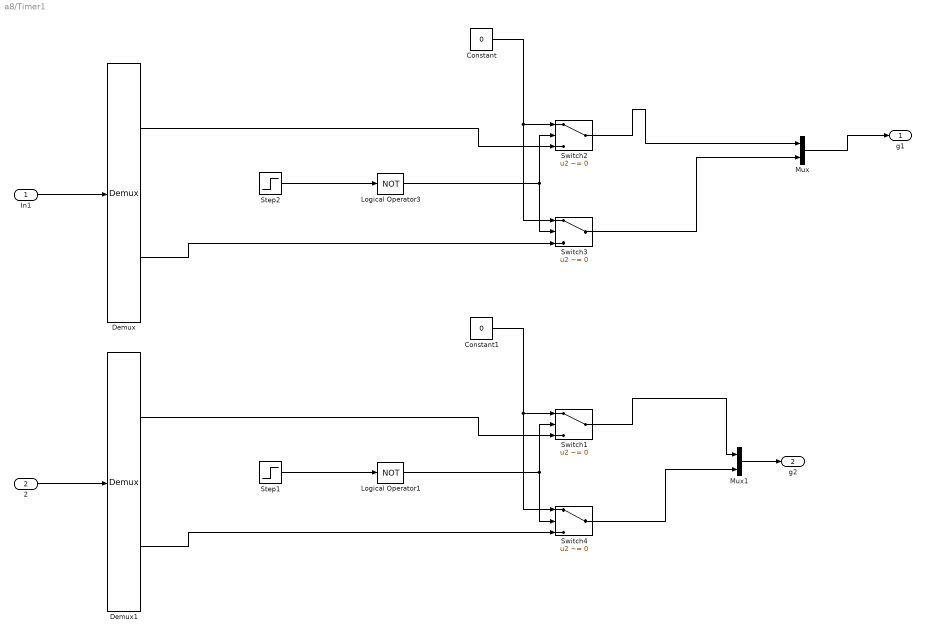
== system a8/Timer1 ==
  In1 : Inport
  2 : Inport  Port=2
  Constant : Constant  Value=0
  Constant1 : Constant  Value=0
  Demux : Demux  Outputs=2
  Demux1 : Demux  Outputs=2
  Logical Operator1 : Logic  Operator=NOT  AllPortsSameDT=off  OutDataTypeStr=boolean
  Logical Operator3 : Logic  Operator=NOT  AllPortsSameDT=off  OutDataTypeStr=boolean
  Mux : Mux  Inputs=2
  Mux1 : Mux  Inputs=2
  Step1 : Step  Time=0  SampleTime=0
  Step2 : Step  Time=0  SampleTime=0
  Switch{1..4} (4 alike) : Switch  Criteria=u2 ~= 0
  g1 : Outport
  g2 : Outport  Port=2
  wires:
  Constant/1 -> Switch3/1, Switch2/1
  Step2/1 -> Logical Operator3/1
  Logical Operator3/1 -> Switch3/2, Switch2/2
  In1/1 -> Demux/1
  Demux/1 -> Switch2/3
  Demux/2 -> Switch3/3
  Switch2/1 -> Mux/1
  Switch3/1 -> Mux/2
  Switch4/1 -> Mux1/2
  Step1/1 -> Logical Operator1/1
  Demux1/2 -> Switch4/3
  2/1 -> Demux1/1
  Switch1/1 -> Mux1/1
  Logical Operator1/1 -> Switch4/2, Switch1/2
  Demux1/1 -> Switch1/3
  Constant1/1 -> Switch4/1, Switch1/1
  Mux/1 -> g1/1
  Mux1/1 -> g2/1

== system a8/Control Algorithm/HSC ==
  isa* : Inport
  isa : Inport  Port=2
  Relay : Relay  OnSwitchValue=h/2  OffSwitchValue=-h/2
  Sum1 : Sum  Inputs=-+  InputSameDT=on  SaturateOnIntegerOverflow=on  OutDataTypeStr=Inherit: Same as first input
  g : Outport  InitialOutput=0
  wires:
  Sum1/1 -> Relay/1
  Relay/1 -> g/1
  isa/1 -> Sum1/1
  isa*/1 -> Sum1/2

== system a8/Control Algorithm/HSC1 ==
  isa* : Inport
  isa : Inport  Port=2
  Relay : Relay  OnSwitchValue=h/2  OffSwitchValue=-h/2
  Sum1 : Sum  Inputs=-+  InputSameDT=on  SaturateOnIntegerOverflow=on  OutDataTypeStr=Inherit: Same as first input
  g : Outport  InitialOutput=0
  wires:
  isa*/1 -> Sum1/2
  isa/1 -> Sum1/1
  Relay/1 -> g/1
  Sum1/1 -> Relay/1

== system a8/Control Algorithm/HSC2 ==
  isa* : Inport
  isa : Inport  Port=2
  Relay : Relay  OnSwitchValue=h/2  OffSwitchValue=-h/2
  Sum1 : Sum  Inputs=-+  InputSameDT=on  SaturateOnIntegerOverflow=on  OutDataTypeStr=Inherit: Same as first input
  g : Outport  InitialOutput=0
  wires:
  Sum1/1 -> Relay/1
  Relay/1 -> g/1
  isa/1 -> Sum1/1
  isa*/1 -> Sum1/2

== system a8/Control Algorithm/HSC3 ==
  isa* : Inport
  isa : Inport  Port=2
  Relay : Relay  OnSwitchValue=h/2  OffSwitchValue=-h/2
  Sum1 : Sum  Inputs=-+  InputSameDT=on  SaturateOnIntegerOverflow=on  OutDataTypeStr=Inherit: Same as first input
  g : Outport  InitialOutput=0
  wires:
  Sum1/1 -> Relay/1
  Relay/1 -> g/1
  isa/1 -> Sum1/1
  isa*/1 -> Sum1/2

== system a8/Control Algorithm/HSC4 ==
  isa* : Inport
  isa : Inport  Port=2
  Relay : Relay  OnSwitchValue=h/2  OffSwitchValue=-h/2
  Sum1 : Sum  Inputs=-+  InputSameDT=on  SaturateOnIntegerOverflow=on  OutDataTypeStr=Inherit: Same as first input
  g : Outport  InitialOutput=0
  wires:
  Sum1/1 -> Relay/1
  Relay/1 -> g/1
  isa/1 -> Sum1/1
  isa*/1 -> Sum1/2

== system a8/Control Algorithm/Self Tuning Filter ==
  a : Inport
  b : Inport  Port=2
  c : Inport  Port=3
  Input : Inport  Port=4
  Subsystem1 : Subsystem
  Subsystem2 : Subsystem
  Subsystem3 : Subsystem
  a1 : Outport
  b1 : Outport  Port=2
  c1 : Outport  Port=3
  wires:
  Subsystem3/1(a1) -> a1/1
  Subsystem1/1(a1) -> b1/1
  Subsystem2/1(a1) -> c1/1
  c/1 -> Subsystem2/1(a)
  b/1 -> Subsystem1/1(a)
  a/1 -> Subsystem3/1(a)
  Input/1 -> Subsystem3/2(Input), Subsystem1/2(Input), Subsystem2/2(Input)

== system a8/Control Algorithm/Subsystem1 ==
  In1 : Inport
  In2 : Inport  Port=2
  Abs : Abs
  Constant5 : Constant  Value=0  VectorParams1D=off
  Data Type Conversion1 : DataTypeConversion  OutDataTypeStr=double  SaturateOnIntegerOverflow=on  RndMeth=Zero
  Relational Operator2 : RelationalOperator  RndMeth=Nearest  InputSameDT=on
  Sample and Hold : dspsigops/Sample and Hold  trig=Either edge  initCond=0  latchinput=off
  Out1 : Outport
  wires:
  In1/1 -> Sample and Hold/1
  Constant5/1 -> Relational Operator2/2
  Relational Operator2/1 -> Data Type Conversion1/1
  In2/1 -> Relational Operator2/1
  Data Type Conversion1/1 -> Sample and Hold/Trigger
  Sample and Hold/1 -> Abs/1
  Abs/1 -> Out1/1

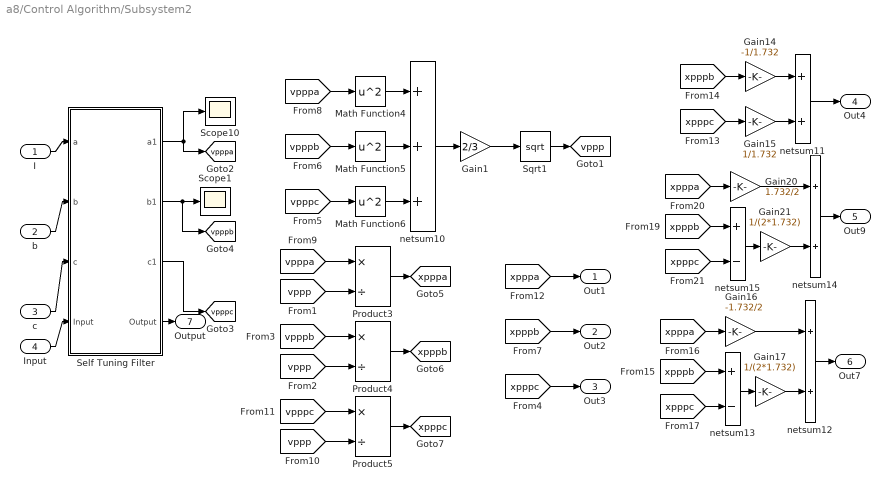
== system a8/Control Algorithm/Subsystem2 ==
  I : Inport
  b : Inport  Port=2
  c : Inport  Port=3
  Input : Inport  Port=4
  Gain1 : Gain  Gain=2/3
  Gain14 : Gain  Gain=-1/1.732
  Gain15 : Gain  Gain=1/1.732
  Gain16 : Gain  Gain=-1.732/2
  Gain17 : Gain  Gain=1/(2*1.732)
  Gain20 : Gain  Gain=1.732/2
  Gain21 : Gain  Gain=1/(2*1.732)
  Math Function4 : Math  Operator=square  SignedPower=on  SaturateOnIntegerOverflow=on
  Math Function5 : Math  Operator=square  SignedPower=on  SaturateOnIntegerOverflow=on
  Math Function6 : Math  Operator=square  SignedPower=on  SaturateOnIntegerOverflow=on
  Product3 : Product  Inputs=*/  RndMeth=Zero
  Product4 : Product  Inputs=*/  RndMeth=Zero
  Product5 : Product  Inputs=*/  RndMeth=Zero
  Scope1 : Scope
  Scope10 : Scope
  Self Tuning Filter : Subsystem
  Sqrt1 : Sqrt  SaturateOnIntegerOverflow=on
  netsum10 : Sum  Inputs=+++  InputSameDT=on  SaturateOnIntegerOverflow=on  OutDataTypeStr=Inherit: Same as first input
  netsum11 : Sum  InputSameDT=on  SaturateOnIntegerOverflow=on  OutDataTypeStr=Inherit: Same as first input
  netsum12 : Sum  InputSameDT=on  SaturateOnIntegerOverflow=on  OutDataTypeStr=Inherit: Same as first input
  netsum13 : Sum  Inputs=+-  InputSameDT=on  SaturateOnIntegerOverflow=on  OutDataTypeStr=Inherit: Same as first input
  netsum14 : Sum  InputSameDT=on  SaturateOnIntegerOverflow=on  OutDataTypeStr=Inherit: Same as first input
  netsum15 : Sum  Inputs=+-  InputSameDT=on  SaturateOnIntegerOverflow=on  OutDataTypeStr=Inherit: Same as first input
  Out1 : Outport
  Out2 : Outport  Port=2
  Out3 : Outport  Port=3
  Out4 : Outport  Port=4
  Out9 : Outport  Port=5
  Out7 : Outport  Port=6
  Output : Outport  Port=7
  tag scope: vppp=global, vpppa=global, vpppb=global, vpppc=global, xpppa=global, xpppb=global, xpppc=global
  wires:
  Math Function4/1 -> netsum10/1
  Math Function5/1 -> netsum10/2
  Math Function6/1 -> netsum10/3
  netsum10/1 -> Gain1/1
  Sqrt1/1 -> [vppp]
  I/1 -> Self Tuning Filter/1(a)
  c/1 -> Self Tuning Filter/3(c)
  b/1 -> Self Tuning Filter/2(b)
  [vpppb] -> Math Function5/1
  [vpppa] -> Math Function4/1
  [vpppc] -> Math Function6/1
  [vpppa] -> Product3/1
  [vppp] -> Product3/2
  [vppp] -> Product4/2
  [vpppb] -> Product4/1
  [vpppc] -> Product5/1
  [vppp] -> Product5/2
  Product3/1 -> [xpppa]
  Product4/1 -> [xpppb]
  Product5/1 -> [xpppc]
  [xpppa] -> Out1/1
  [xpppb] -> Out2/1
  [xpppc] -> Out3/1
  [xpppb] -> Gain14/1
  Gain14/1 -> netsum11/1
  Gain15/1 -> netsum11/2
  [xpppc] -> Gain15/1
  netsum11/1 -> Out4/1
  netsum14/1 -> Out9/1
  [xpppb] -> netsum15/1
  Gain21/1 -> netsum14/2
  Gain20/1 -> netsum14/1
  [xpppa] -> Gain20/1
  [xpppc] -> netsum15/2
  netsum15/1 -> Gain21/1
  netsum13/1 -> Gain17/1
  [xpppc] -> netsum13/2
  [xpppa] -> Gain16/1
  Gain16/1 -> netsum12/1
  Gain17/1 -> netsum12/2
  [xpppb] -> netsum13/1
  netsum12/1 -> Out7/1
  Gain1/1 -> Sqrt1/1
  Self Tuning Filter/1(a1) -> [vpppa], Scope10/1
  Self Tuning Filter/2(b1) -> [vpppb], Scope1/1
  Self Tuning Filter/3(c1) -> [vpppc]
  Input/1 -> Self Tuning Filter/4(Input)
  Self Tuning Filter/4(Output) -> Output/1

== system a8/Control Algorithm/Subsystem3 ==
  In1 : Inport
  Add : Sum
  Gain : Gain
  Gain1 : Gain  Gain=10
  Integrator : Integrator  ZeroCross=off
  Out1 : Outport
  wires:
  Gain1/1 -> Integrator/1
  Gain/1 -> Add/1
  Add/1 -> Out1/1
  Integrator/1 -> Add/2
  In1/1 -> Gain/1, Gain1/1

== system a8/Control Algorithm/Subsystem4 ==
  In1 : Inport
  Add : Sum
  Gain : Gain
  Gain1 : Gain  Gain=2
  Integrator : Integrator  ZeroCross=off
  Out1 : Outport
  wires:
  In1/1 -> Gain/1, Gain1/1
  Gain1/1 -> Integrator/1
  Gain/1 -> Add/1
  Add/1 -> Out1/1
  Integrator/1 -> Add/2

== system a8/Control Algorithm/Subsystem5 ==
  b1 : Inport
  In2 : Inport  Port=2
  Abs : Abs
  Constant5 : Constant  Value=0  VectorParams1D=off
  Data Type Conversion1 : DataTypeConversion  OutDataTypeStr=double  SaturateOnIntegerOverflow=on  RndMeth=Zero
  Relational Operator2 : RelationalOperator  RndMeth=Nearest  InputSameDT=on
  Sample and Hold : dspsigops/Sample and Hold  trig=Either edge  initCond=0  latchinput=off
  Out1 : Outport
  wires:
  b1/1 -> Sample and Hold/1
  Constant5/1 -> Relational Operator2/2
  Relational Operator2/1 -> Data Type Conversion1/1
  In2/1 -> Relational Operator2/1
  Data Type Conversion1/1 -> Sample and Hold/Trigger
  Sample and Hold/1 -> Abs/1
  Abs/1 -> Out1/1

== system a8/Control Algorithm/Subsystem6 ==
  b1 : Inport
  In2 : Inport  Port=2
  Abs : Abs
  Constant5 : Constant  Value=0  VectorParams1D=off
  Data Type Conversion1 : DataTypeConversion  OutDataTypeStr=double  SaturateOnIntegerOverflow=on  RndMeth=Zero
  Relational Operator2 : RelationalOperator  RndMeth=Nearest  InputSameDT=on
  Sample and Hold : dspsigops/Sample and Hold  trig=Either edge  initCond=0  latchinput=off
  Out1 : Outport
  wires:
  b1/1 -> Sample and Hold/1
  Constant5/1 -> Relational Operator2/2
  Relational Operator2/1 -> Data Type Conversion1/1
  In2/1 -> Relational Operator2/1
  Data Type Conversion1/1 -> Sample and Hold/Trigger
  Sample and Hold/1 -> Abs/1
  Abs/1 -> Out1/1

== system a8/Control Algorithm/Self Tuning Filter/Subsystem1 ==
  a : Inport
  Input : Inport  Port=2
  Gain : Gain  Gain=70.71
  Integrator : Integrator
  Integrator1 : Integrator
  Product : Product
  Product1 : Product
  Scope1 : Scope
  Scope2 : Scope
  Sum : Sum  Inputs=-+
  Sum1 : Sum  Inputs=|+-
  a1 : Outport
  wires:
  Sum/1 -> Gain/1
  a/1 -> Scope1/1, Sum/2
  Integrator/1 -> Scope2/1, a1/1, Sum/1, Product/1
  Gain/1 -> Sum1/1
  Integrator1/1 -> Product1/1
  Sum1/1 -> Integrator/1
  Product/1 -> Integrator1/1
  Product1/1 -> Sum1/2
  Input/1 -> Product1/2, Product/2

== system a8/Control Algorithm/Self Tuning Filter/Subsystem2 ==
  a : Inport
  Input : Inport  Port=2
  Gain : Gain  Gain=70.71
  Integrator : Integrator
  Integrator1 : Integrator
  Product : Product
  Product1 : Product
  Scope1 : Scope
  Scope2 : Scope
  Sum : Sum  Inputs=-+
  Sum1 : Sum  Inputs=|+-
  a1 : Outport
  wires:
  Sum/1 -> Gain/1
  a/1 -> Scope1/1, Sum/2
  Integrator/1 -> Scope2/1, a1/1, Sum/1, Product/1
  Gain/1 -> Sum1/1
  Integrator1/1 -> Product1/1
  Sum1/1 -> Integrator/1
  Product/1 -> Integrator1/1
  Product1/1 -> Sum1/2
  Input/1 -> Product1/2, Product/2

== system a8/Control Algorithm/Self Tuning Filter/Subsystem3 ==
  a : Inport
  Input : Inport  Port=2
  Gain : Gain  Gain=70.71
  Integrator : Integrator
  Integrator1 : Integrator
  Product : Product
  Product1 : Product
  Scope1 : Scope
  Scope2 : Scope
  Sum : Sum  Inputs=-+
  Sum1 : Sum  Inputs=|+-
  a1 : Outport
  wires:
  Sum/1 -> Gain/1
  a/1 -> Scope1/1, Sum/2
  Integrator/1 -> Scope2/1, a1/1, Sum/1, Product/1
  Gain/1 -> Sum1/1
  Integrator1/1 -> Product1/1
  Sum1/1 -> Integrator/1
  Product/1 -> Integrator1/1
  Product1/1 -> Sum1/2
  Input/1 -> Product/2, Product1/2

== system a8/Control Algorithm/Subsystem2/Self Tuning Filter ==
  a : Inport
  b : Inport  Port=2
  c : Inport  Port=3
  Input : Inport  Port=4
  Subsystem1 : Subsystem
  Subsystem2 : Subsystem
  Subsystem3 : Subsystem
  a1 : Outport
  b1 : Outport  Port=2
  c1 : Outport  Port=3
  Output : Outport  Port=4
  wires:
  Subsystem2/1(a1) -> a1/1
  Subsystem1/1(a1) -> b1/1
  Subsystem3/1(a1) -> c1/1
  c/1 -> Subsystem3/1(a)
  b/1 -> Subsystem1/1(a)
  a/1 -> Subsystem2/1(a)
  Input/1 -> Subsystem2/2(Input), Subsystem3/2(Input), Subsystem1/2(Input)
  Subsystem2/2(Output) -> Output/1

== system a8/Control Algorithm/Subsystem2/Self Tuning Filter/Subsystem1 ==
  a : Inport
  Input : Inport  Port=2
  Gain : Gain  Gain=70.71
  Integrator : Integrator  UpperSaturationLimit=200  LowerSaturationLimit=-200
  Integrator1 : Integrator
  Product : Product
  Product1 : Product
  Scope : Scope
  Scope1 : Scope
  Scope2 : Scope
  Subsystem : Subsystem
  Sum : Sum  Inputs=-+
  Sum1 : Sum  Inputs=|+-
  a1 : Outport
  wires:
  Sum/1 -> Gain/1
  a/1 -> Subsystem/1(In1), Scope1/1, Sum/2
  Integrator/1 -> Scope2/1, a1/1, Sum/1, Product/1
  Gain/1 -> Sum1/1
  Integrator1/1 -> Product1/1
  Sum1/1 -> Integrator/1
  Product/1 -> Integrator1/1
  Product1/1 -> Sum1/2
  Input/1 -> Subsystem/2(Input)
  Subsystem/1(Output) -> Product/2, Product1/2, Scope/1

== system a8/Control Algorithm/Subsystem2/Self Tuning Filter/Subsystem2 ==
  a : Inport
  Input : Inport  Port=2
  Gain : Gain  Gain=70.71
  Integrator : Integrator  UpperSaturationLimit=200  LowerSaturationLimit=-200
  Integrator1 : Integrator
  Product : Product
  Product1 : Product
  Scope : Scope
  Scope1 : Scope
  Scope2 : Scope
  Subsystem : Subsystem
  Sum : Sum  Inputs=-+
  Sum1 : Sum  Inputs=|+-
  a1 : Outport
  Output : Outport  Port=2
  wires:
  Sum/1 -> Gain/1
  a/1 -> Subsystem/1(In1), Scope1/1, Sum/2
  Integrator/1 -> Scope2/1, a1/1, Sum/1, Product/1
  Gain/1 -> Sum1/1
  Integrator1/1 -> Product1/1
  Sum1/1 -> Integrator/1
  Product/1 -> Integrator1/1
  Product1/1 -> Sum1/2
  Input/1 -> Subsystem/2(Input)
  Subsystem/1(Output) -> Output/1, Product/2, Product1/2, Scope/1

== system a8/Control Algorithm/Subsystem2/Self Tuning Filter/Subsystem3 ==
  a : Inport
  Input : Inport  Port=2
  Gain : Gain  Gain=70.71
  Integrator : Integrator  UpperSaturationLimit=200  LowerSaturationLimit=-200
  Integrator1 : Integrator
  Product : Product
  Product1 : Product
  Scope : Scope
  Scope1 : Scope
  Scope2 : Scope
  Subsystem : Subsystem
  Sum : Sum  Inputs=-+
  Sum1 : Sum  Inputs=|+-
  a1 : Outport
  wires:
  Sum/1 -> Gain/1
  a/1 -> Subsystem/1(In1), Scope1/1, Sum/2
  Integrator/1 -> Scope2/1, a1/1, Sum/1, Product/1
  Gain/1 -> Sum1/1
  Integrator1/1 -> Product1/1
  Sum1/1 -> Integrator/1
  Product/1 -> Integrator1/1
  Product1/1 -> Sum1/2
  Input/1 -> Subsystem/2(Input)
  Subsystem/1(Output) -> Product/2, Product1/2, Scope/1

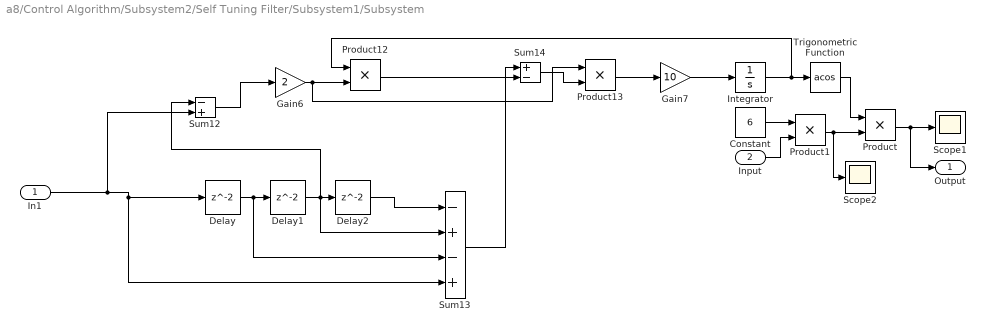
== system a8/Control Algorithm/Subsystem2/Self Tuning Filter/Subsystem1/Subsystem ==
  In1 : Inport
  Input : Inport  Port=2
  Constant : Constant  Value=6
  Delay : Delay
  Delay1 : Delay
  Delay2 : Delay
  Gain6 : Gain  Gain=2
  Gain7 : Gain  Gain=10
  Integrator : Integrator
  Product{,1,12..13} (4 alike) : Product
  Scope1 : Scope
  Scope2 : Scope
  Sum12 : Sum  Inputs=-+
  Sum13 : Sum  Inputs=-+-+
  Sum14 : Sum  Inputs=+-
  Trigonometric Function : Trigonometry  Operator=acos  RemoveProtectionAgainstOutOfRangeInput=on
  Output : Outport
  wires:
  In1/1 -> Sum13/4, Delay/1, Sum12/2
  Sum13/1 -> Sum14/1
  Sum14/1 -> Product13/2
  Gain6/1 -> Product13/1, Product12/2
  Delay2/1 -> Sum13/1
  Product12/1 -> Sum14/2
  Integrator/1 -> Product12/1, Trigonometric Function/1
  Delay/1 -> Sum13/3, Delay1/1
  Trigonometric Function/1 -> Product/1
  Gain7/1 -> Integrator/1
  Sum12/1 -> Gain6/1
  Product13/1 -> Gain7/1
  Delay1/1 -> Sum12/1, Sum13/2, Delay2/1
  Product1/1 -> Scope2/1, Product/2
  Product/1 -> Output/1, Scope1/1
  Constant/1 -> Product1/1
  Input/1 -> Product1/2

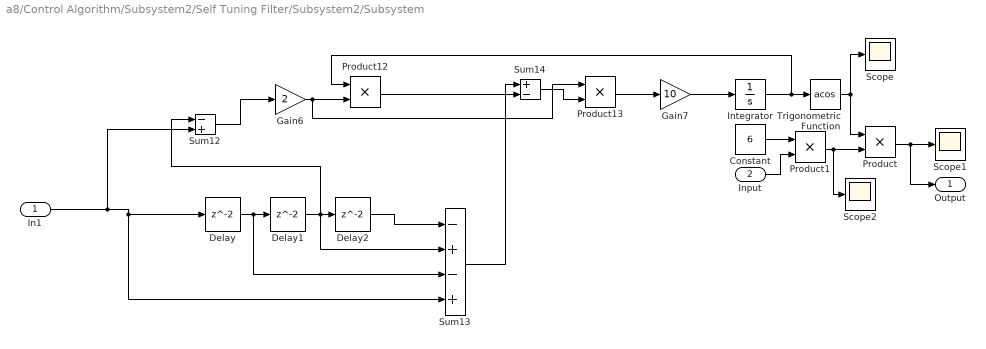
== system a8/Control Algorithm/Subsystem2/Self Tuning Filter/Subsystem2/Subsystem ==
  In1 : Inport
  Input : Inport  Port=2
  Constant : Constant  Value=6
  Delay : Delay
  Delay1 : Delay
  Delay2 : Delay
  Gain6 : Gain  Gain=2
  Gain7 : Gain  Gain=10
  Integrator : Integrator
  Product{,1,12..13} (4 alike) : Product
  Scope : Scope
  Scope1 : Scope
  Scope2 : Scope
  Sum12 : Sum  Inputs=-+
  Sum13 : Sum  Inputs=-+-+
  Sum14 : Sum  Inputs=+-
  Trigonometric Function : Trigonometry  Operator=acos  RemoveProtectionAgainstOutOfRangeInput=on
  Output : Outport
  wires:
  In1/1 -> Sum13/4, Delay/1, Sum12/2
  Sum13/1 -> Sum14/1
  Sum14/1 -> Product13/2
  Gain6/1 -> Product13/1, Product12/2
  Delay2/1 -> Sum13/1
  Product12/1 -> Sum14/2
  Integrator/1 -> Product12/1, Trigonometric Function/1
  Delay/1 -> Sum13/3, Delay1/1
  Gain7/1 -> Integrator/1
  Sum12/1 -> Gain6/1
  Product13/1 -> Gain7/1
  Delay1/1 -> Sum12/1, Sum13/2, Delay2/1
  Product1/1 -> Scope2/1, Product/2
  Product/1 -> Output/1, Scope1/1
  Constant/1 -> Product1/1
  Input/1 -> Product1/2
  Trigonometric Function/1 -> Product/1, Scope/1

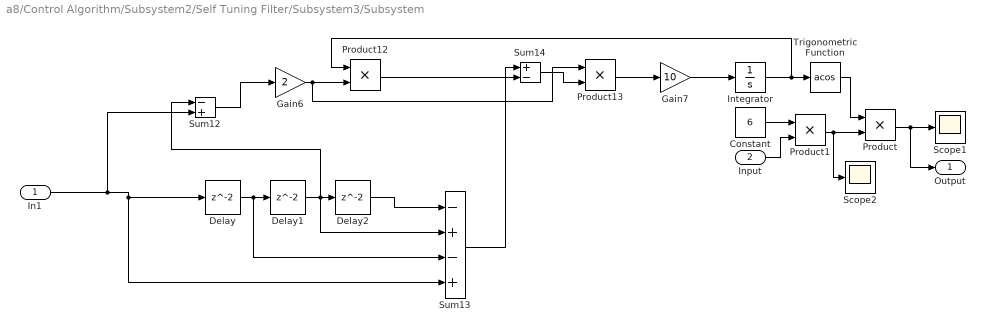
== system a8/Control Algorithm/Subsystem2/Self Tuning Filter/Subsystem3/Subsystem ==
  In1 : Inport
  Input : Inport  Port=2
  Constant : Constant  Value=6
  Delay : Delay
  Delay1 : Delay
  Delay2 : Delay
  Gain6 : Gain  Gain=2
  Gain7 : Gain  Gain=10
  Integrator : Integrator
  Product{,1,12..13} (4 alike) : Product
  Scope1 : Scope
  Scope2 : Scope
  Sum12 : Sum  Inputs=-+
  Sum13 : Sum  Inputs=-+-+
  Sum14 : Sum  Inputs=+-
  Trigonometric Function : Trigonometry  Operator=acos  RemoveProtectionAgainstOutOfRangeInput=on
  Output : Outport
  wires:
  In1/1 -> Sum13/4, Delay/1, Sum12/2
  Sum13/1 -> Sum14/1
  Sum14/1 -> Product13/2
  Gain6/1 -> Product13/1, Product12/2
  Delay2/1 -> Sum13/1
  Product12/1 -> Sum14/2
  Integrator/1 -> Product12/1, Trigonometric Function/1
  Delay/1 -> Sum13/3, Delay1/1
  Trigonometric Function/1 -> Product/1
  Gain7/1 -> Integrator/1
  Sum12/1 -> Gain6/1
  Product13/1 -> Gain7/1
  Delay1/1 -> Sum12/1, Sum13/2, Delay2/1
  Product1/1 -> Scope2/1, Product/2
  Product/1 -> Output/1, Scope1/1
  Constant/1 -> Product1/1
  Input/1 -> Product1/2
